simulink model "model"  (R2014a)
settings: Solver=ode45  StartTime=0.0  StopTime=2  RelTol=1e-3
libraries: simulink x3, dspsigattribs x2, dspinverses x1
settings Model: Creator=Lauszus  LastModifiedBy=Lauszus

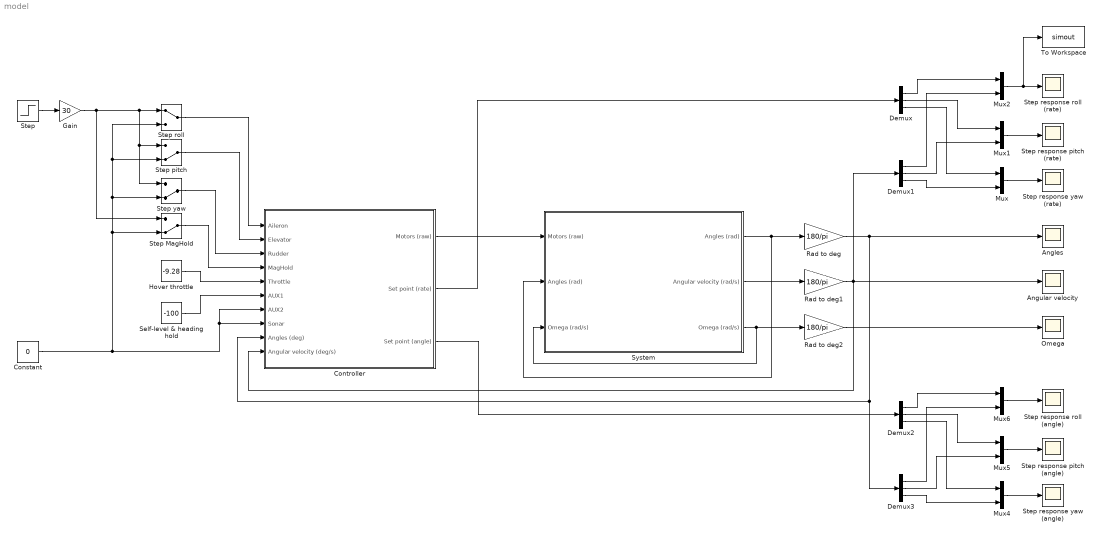
== system model ==
  Angles : Scope
      settings: SaveName=ScopeData2  MaxDataPoints=100000
  Angular velocity : Scope
      settings: MaxDataPoints=100000
  Constant : Constant  Value=0
  Controller : Subsystem
  Demux{,1..3} (4 alike) : Demux  Outputs=3
  Gain : Gain  Gain=30
  Hover throttle : Constant  Value=-9.28
  Mux{,1..2,4..6} (6 alike) : Mux  Inputs=2
  Omega : Scope
      settings: YMin=-2.5  YMax=47.5  SaveName=ScopeData3  MaxDataPoints=100000
  Rad to deg : Gain  Gain=180/pi
  Rad to deg1 : Gain  Gain=180/pi
  Rad to deg2 : Gain  Gain=180/pi
  Self-level & heading hold : Constant  Value=-100
  Step : Step  SampleTime=0
  Step MagHold : ManualSwitch  CurrentSetting=0
  Step pitch : ManualSwitch  CurrentSetting=0
  Step response pitch (angle) : Scope
      settings: SaveName=ScopeData4  MaxDataPoints=100000
  Step response pitch (rate) : Scope
      settings: YMin=46.9  YMax=46.9001  SaveName=ScopeData6  MaxDataPoints=100000
  Step response roll (angle) : Scope
      settings: YMin=44  YMax=48.25  SaveName=ScopeData5  MaxDataPoints=100000
  Step response roll (rate) : Scope
      settings: YMin=44  YMax=48.25  SaveName=ScopeData11  MaxDataPoints=100000
  Step response yaw (angle) : Scope
      settings: YMin=19  YMax=21  SaveName=ScopeData7  MaxDataPoints=100000
  Step response yaw (rate) : Scope
      settings: YMin=19  YMax=21  SaveName=ScopeData10  MaxDataPoints=100000
  Step roll : ManualSwitch
  Step yaw : ManualSwitch  CurrentSetting=0
  System : Subsystem
  To Workspace : ToWorkspace  VariableName=simout  SaveFormat=Timeseries  SampleTime=-1
  wires:
  Self-level & heading hold/1 -> Controller/6(AUX1)
  Constant/1 -> Step MagHold/2, Step pitch/2, Step roll/2, Step yaw/2, Controller/8(Sonar), Controller/7(AUX2)
  Hover throttle/1 -> Controller/5(Throttle)
  System/2(Angular velocity (rad/s)) -> Rad to deg1/1
  Controller/2(Set point (rate)) -> Demux/1
  Step roll/1 -> Controller/1(Aileron)
  Step pitch/1 -> Controller/2(Elevator)
  Mux/1 -> Step response yaw (rate)/1
  Mux1/1 -> Step response pitch (rate)/1
  Mux2/1 -> To Workspace/1, Step response roll (rate)/1
  Demux1/3 -> Mux/2
  Demux/1 -> Mux2/1
  Demux/2 -> Mux1/1
  Demux/3 -> Mux/1
  Demux1/1 -> Mux2/2
  Demux1/2 -> Mux1/2
  Step yaw/1 -> Controller/3(Rudder)
  Step MagHold/1 -> Controller/4(MagHold)
  Step/1 -> Gain/1
  Controller/1(Motors (raw)) -> System/1(Motors (raw))
  System/1(Angles (rad)) -> Rad to deg/1, System/2("Angles (rad) ")
  Gain/1 -> Step yaw/1, Step pitch/1, Step roll/1, Step MagHold/1
  System/3(Omega (rad/s)) -> Rad to deg2/1, System/3("Omega (rad/s) ")
  Rad to deg1/1 -> Controller/10(Angular velocity (deg/s)), Demux1/1, Angular velocity/1
  Rad to deg/1 -> Demux3/1, Controller/9(Angles (deg)), Angles/1
  Rad to deg2/1 -> Omega/1
  Mux5/1 -> Step response pitch (angle)/1
  Mux6/1 -> Step response roll (angle)/1
  Demux3/3 -> Mux4/2
  Demux2/1 -> Mux6/1
  Demux2/2 -> Mux5/1
  Demux2/3 -> Mux4/1
  Demux3/2 -> Mux5/2
  Controller/3(Set point (angle)) -> Demux2/1
  Demux3/1 -> Mux6/2
  Mux4/1 -> Step response yaw (angle)/1

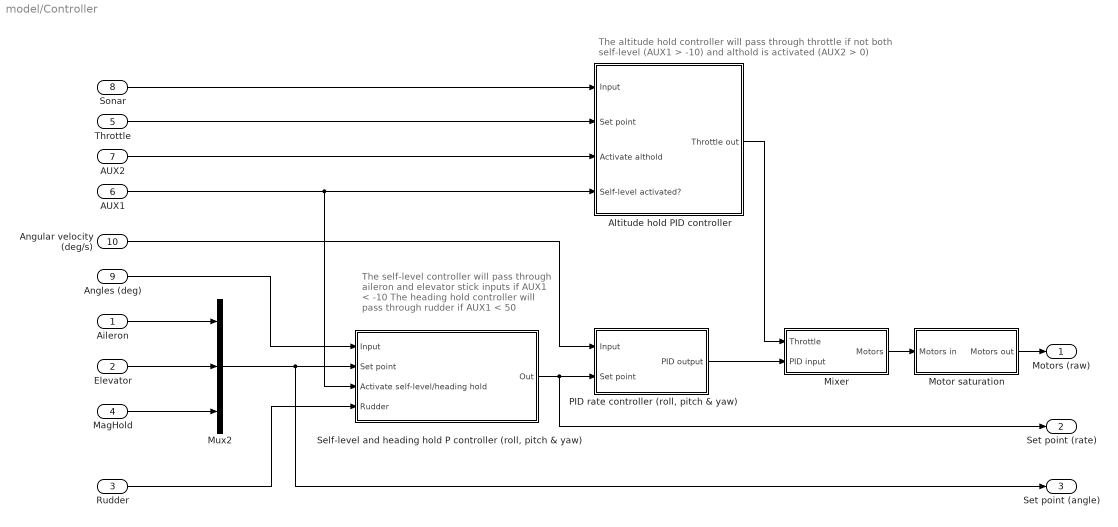
== system model/Controller ==
  note: The self-level controller will pass through aileron and elevator stick inputs if AUX1 < -10
      | The heading hold controller will pass through rudder if AUX1 < 50
  note: The altitude hold controller will pass through throttle if not both
      | self-level (AUX1 > -10) and althold is activated (AUX2 > 0)
  Aileron : Inport
  Elevator : Inport  Port=2
  Rudder : Inport  Port=3
  MagHold : Inport  Port=4
  Throttle : Inport  Port=5
  AUX1 : Inport  Port=6
  AUX2 : Inport  Port=7
  Sonar : Inport  Port=8
  Angles (deg) : Inport  Port=9
  Angular velocity (deg/s) : Inport  Port=10
  Altitude hold PID controller : Subsystem
  Mixer : Subsystem
  Motor saturation : Subsystem
  Mux2 : Mux  Inputs=3
  "PID rate controller (roll, pitch & yaw)" : Subsystem
  "Self-level and heading hold P controller (roll, pitch & yaw)" : Subsystem
  Motors (raw) : Outport
  Set point (rate) : Outport  Port=2
  Set point (angle) : Outport  Port=3
  wires:
  AUX1/1 -> "Self-level and heading hold P controller (roll, pitch & yaw)"/3(Activate self-level/heading hold), Altitude hold PID controller/4(Self-level activated?)
  Angular velocity (deg/s)/1 -> "PID rate controller (roll, pitch & yaw)"/1(Input)
  "Self-level and heading hold P controller (roll, pitch & yaw)"/1(Out) -> "PID rate controller (roll, pitch & yaw)"/2(Set point), Set point (rate)/1
  Sonar/1 -> Altitude hold PID controller/1(Input)
  Throttle/1 -> Altitude hold PID controller/2(Set point)
  AUX2/1 -> Altitude hold PID controller/3(Activate althold)
  Altitude hold PID controller/1(Throttle out) -> Mixer/1(Throttle)
  "PID rate controller (roll, pitch & yaw)"/1(PID output) -> Mixer/2(PID input)
  Mixer/1(Motors) -> Motor saturation/1(Motors in)
  Motor saturation/1(Motors out) -> Motors (raw)/1
  Angles (deg)/1 -> "Self-level and heading hold P controller (roll, pitch & yaw)"/1(Input)
  Aileron/1 -> Mux2/1
  Elevator/1 -> Mux2/2
  Mux2/1 -> Set point (angle)/1, "Self-level and heading hold P controller (roll, pitch & yaw)"/2(Set point)
  MagHold/1 -> Mux2/3
  Rudder/1 -> "Self-level and heading hold P controller (roll, pitch & yaw)"/4(Rudder)

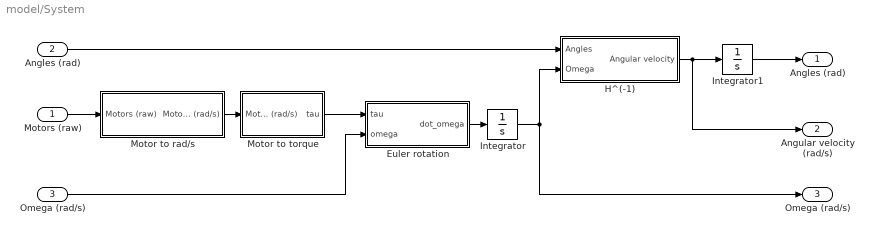
== system model/System ==
  Motors (raw) : Inport
  "Angles (rad) " : Inport  Port=2
  "Omega (rad/s) " : Inport  Port=3
  Euler rotation : Subsystem
  H^(-1) : Subsystem
  Integrator : Integrator
  Integrator1 : Integrator
  Motor to rad/s : Subsystem
  Motor to torque : Subsystem
  Angles (rad) : Outport
  Angular velocity (rad/s) : Outport  Port=2
  Omega (rad/s) : Outport  Port=3
  wires:
  Integrator1/1 -> Angles (rad)/1
  "Angles (rad) "/1 -> H^(-1)/1("Angles ")
  Integrator/1 -> Omega (rad/s)/1, H^(-1)/2(Omega)
  "Omega (rad/s) "/1 -> Euler rotation/2(omega)
  Euler rotation/1(dot_omega) -> Integrator/1
  Motor to torque/1(tau) -> Euler rotation/1(tau)
  Motor to rad/s/1(Motors (rad/s)) -> Motor to torque/1(Motors (rad/s))
  Motors (raw)/1 -> Motor to rad/s/1(Motors (raw))
  H^(-1)/1(Angular velocity) -> Integrator1/1, Angular velocity (rad/s)/1

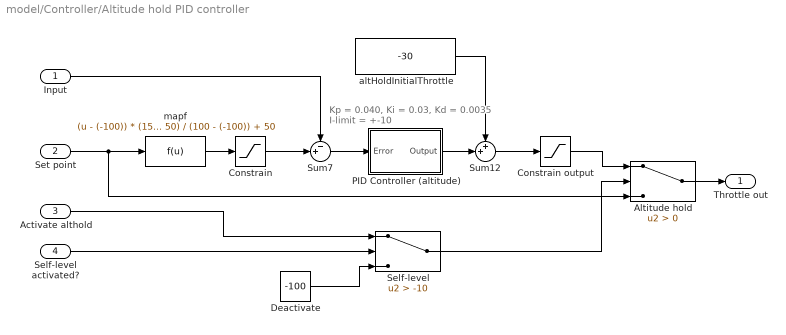
== system model/Controller/Altitude hold PID controller ==
  note: Kp = 0.040, Ki = 0.03, Kd = 0.0035
      | I-limit =  +-10
  Input : Inport
  Set point : Inport  Port=2
  Activate althold : Inport  Port=3
  Self-level activated? : Inport  Port=4
  Altitude hold : Switch  Criteria=u2 > Threshold
  Constrain : Saturate  UpperLimit=1500  LowerLimit=50
  Constrain output : Saturate  UpperLimit=100  LowerLimit=-90
  Deactivate : Constant  Value=-100
  PID Controller (altitude) : Subsystem
  Self-level : Switch  Criteria=u2 > Threshold  Threshold=-10
  Sum12 : Sum  Inputs=++|
  Sum7 : Sum  Inputs=-+|
  altHoldInitialThrottle : Constant  Value=-30
  mapf : Fcn  Expr=(u - (-100)) * (1500 - 50) / (100 - (-100)) + 50
  Throttle out : Outport
  wires:
  Set point/1 -> mapf/1, Altitude hold/3
  Self-level/1 -> Altitude hold/2
  altHoldInitialThrottle/1 -> Sum12/1
  Sum12/1 -> Constrain output/1
  Constrain output/1 -> Altitude hold/1
  Activate althold/1 -> Self-level/1
  Deactivate/1 -> Self-level/3
  Self-level activated?/1 -> Self-level/2
  mapf/1 -> Constrain/1
  Constrain/1 -> Sum7/2
  Input/1 -> Sum7/1
  Altitude hold/1 -> Throttle out/1
  Sum7/1 -> PID Controller (altitude)/1(Error)
  PID Controller (altitude)/1(Output) -> Sum12/2

== system model/Controller/Mixer ==
  note: Motor 1 is bottom right
      | Motor 2 is top right
      | Motor 3 is bottom left
      | Motor 4 is top left
  Throttle : Inport
  PID input : Inport  Port=2
  Demux : Demux  Outputs=3
  Mux1 : Mux
  Sum : Sum  Inputs=+-+-
  Sum1 : Sum  Inputs=+--+
  Sum2 : Sum  Inputs=++++
  Sum3 : Sum  Inputs=++--
  Motors : Outport
  wires:
  Throttle/1 -> Sum3/1, Sum2/1, Sum1/1, Sum/1
  Demux/2 -> Sum/3, Sum1/3, Sum2/3, Sum3/3
  Demux/3 -> Sum/4, Sum1/4, Sum2/4, Sum3/4
  Demux/1 -> Sum3/2, Sum/2, Sum1/2, Sum2/2
  Sum/1 -> Mux1/1
  Sum1/1 -> Mux1/2
  Sum2/1 -> Mux1/3
  Sum3/1 -> Mux1/4
  Mux1/1 -> Motors/1
  PID input/1 -> Demux/1

== system model/Controller/Motor saturation ==
  Motors in : Inport
  If : If  NumInputs=2  IfExpression=u2 > u1
  Max output : Constant  Value=100
  Merge : Merge
  MinMax : MinMax  Function=max
  Passthrough : Subsystem  TreatAsAtomicUnit=on
  Subtract difference : Subsystem  TreatAsAtomicUnit=on
  Sum13 : Sum  Inputs=-+|
  Motors out : Outport
  wires:
  Motors in/1 -> Subtract difference/2(Motors), Passthrough/1(In1), MinMax/1
  If/1 -> Subtract difference/Action
  Subtract difference/1(Out1) -> Merge/1
  If/2 -> Passthrough/Action
  Passthrough/1(Out1) -> Merge/2
  Max output/1 -> Sum13/1, If/1
  MinMax/1 -> If/2, Sum13/2
  Sum13/1 -> Subtract difference/1(Difference)
  Merge/1 -> Motors out/1

== system model/Controller/PID rate controller (roll, pitch & yaw) ==
  note: Kp = 0.310, Ki = 1.65, Kd = 0.00040
      | I-limit =  +-5.85
  note: Kp = 1, Ki = 6, Kd = 0.00040
      | I-limit =  +-10
  note: Kp = 0.310, Ki = 1.65, Kd = 0.00040
      | I-limit =  +-5.85
  Input : Inport
  Set point : Inport  Port=2
  Demux1 : Demux  Outputs=3
  Mux : Mux  Inputs=3
  PID Controller (pitch) : Subsystem
  PID Controller (roll) : Subsystem
  PID Controller (yaw) : Subsystem
  Sum10 : Sum  Inputs=-+|
  PID output : Outport
  wires:
  Mux/1 -> PID output/1
  Set point/1 -> Sum10/2
  Sum10/1 -> Demux1/1
  Input/1 -> Sum10/1
  Demux1/1 -> PID Controller (roll)/1(Error)
  Demux1/2 -> PID Controller (pitch)/1(Error)
  PID Controller (roll)/1(Output) -> Mux/1
  PID Controller (pitch)/1(Output) -> Mux/2
  Demux1/3 -> PID Controller (yaw)/1(Error)
  PID Controller (yaw)/1(Output) -> Mux/3

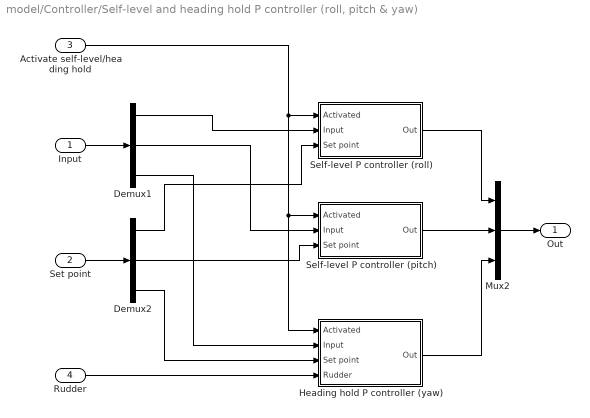
== system model/Controller/Self-level and heading hold P controller (roll, pitch & yaw) ==
  Input : Inport
  Set point : Inport  Port=2
  Activate self-level/heading hold : Inport  Port=3
  Rudder : Inport  Port=4
  Demux1 : Demux  Outputs=3
  Demux2 : Demux  Outputs=3
  Heading hold P controller (yaw) : Subsystem
  Mux2 : Mux  Inputs=3
  Self-level P controller (pitch) : Subsystem
  Self-level P controller (roll) : Subsystem
  Out : Outport
  wires:
  Self-level P controller (roll)/1(Out) -> Mux2/1
  Self-level P controller (pitch)/1(Out) -> Mux2/2
  Input/1 -> Demux1/1
  Set point/1 -> Demux2/1
  Mux2/1 -> Out/1
  Activate self-level/heading hold/1 -> Heading hold P controller (yaw)/1(Activated), Self-level P controller (pitch)/1(Activated), Self-level P controller (roll)/1(Activated)
  Rudder/1 -> Heading hold P controller (yaw)/4(Rudder)
  Heading hold P controller (yaw)/1(Out) -> Mux2/3
  Demux1/1 -> Self-level P controller (roll)/2(Input)
  Demux1/2 -> Self-level P controller (pitch)/2(Input)
  Demux1/3 -> Heading hold P controller (yaw)/2(Input)
  Demux2/1 -> Self-level P controller (roll)/3(Set point)
  Demux2/2 -> Self-level P controller (pitch)/3(Set point)
  Demux2/3 -> Heading hold P controller (yaw)/3(Set point)

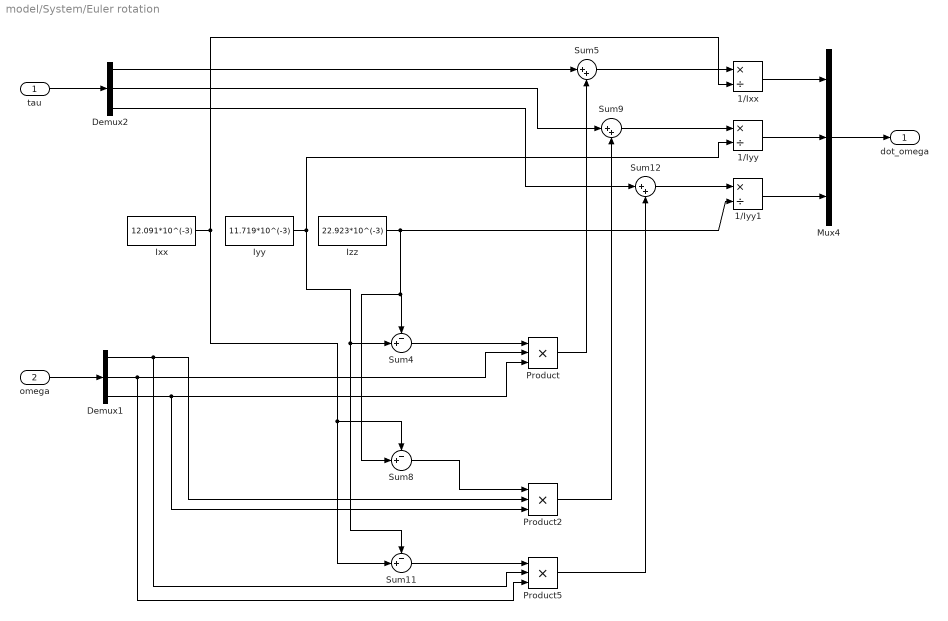
== system model/System/Euler rotation ==
  tau : Inport
  omega : Inport  Port=2
  1/Ixx : Product  Inputs=*/
  1/Iyy : Product  Inputs=*/
  1/Iyy1 : Product  Inputs=*/
  Demux1 : Demux  Outputs=3
  Demux2 : Demux  Outputs=3
  Ixx : Constant  Value=12.091*10^(-3)
  Iyy : Constant  Value=11.719*10^(-3)
  Izz : Constant  Value=22.923*10^(-3)
  Mux4 : Mux  Inputs=3
  Product : Product  Inputs=3
  Product2 : Product  Inputs=3
  Product5 : Product  Inputs=3
  Sum11 : Sum  Inputs=-+|
  Sum12 : Sum  Inputs=|++
  Sum4 : Sum  Inputs=-+|
  Sum5 : Sum  Inputs=|++
  Sum8 : Sum  Inputs=-+|
  Sum9 : Sum  Inputs=|++
  dot_omega : Outport
  wires:
  Iyy/1 -> Sum11/1, Sum4/2, 1/Iyy/2
  Izz/1 -> Sum8/2, Sum4/1, 1/Iyy1/2
  omega/1 -> Demux1/1
  Sum4/1 -> Product/1
  Ixx/1 -> 1/Ixx/2, Sum11/2, Sum8/1
  Sum8/1 -> Product2/1
  Demux1/1 -> Product5/2, Product2/2
  Demux1/2 -> Product5/3, Product/2
  Demux1/3 -> Product2/3, Product/3
  Sum11/1 -> Product5/1
  Mux4/1 -> dot_omega/1
  Sum5/1 -> 1/Ixx/1
  tau/1 -> Demux2/1
  Demux2/1 -> Sum5/1
  Demux2/2 -> Sum9/1
  Demux2/3 -> Sum12/1
  1/Ixx/1 -> Mux4/1
  Sum9/1 -> 1/Iyy/1
  Sum12/1 -> 1/Iyy1/1
  1/Iyy/1 -> Mux4/2
  1/Iyy1/1 -> Mux4/3
  Product/1 -> Sum5/2
  Product2/1 -> Sum9/2
  Product5/1 -> Sum12/2

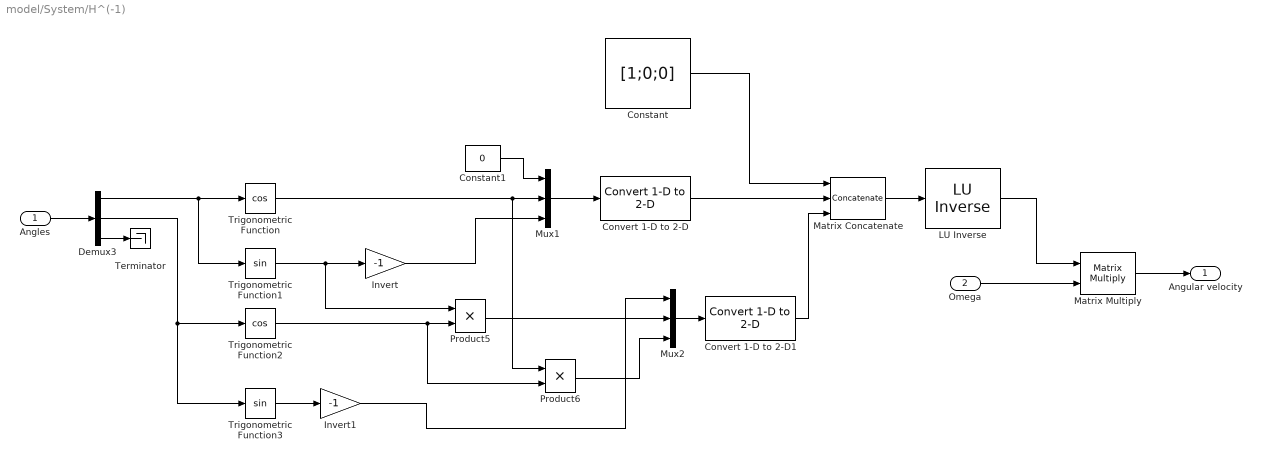
== system model/System/H^(-1) ==
  "Angles " : Inport
  Omega : Inport  Port=2
  " LU Inverse" : dspinverses/ LU Inverse
  Constant : Constant  Value=[1;0;0]  VectorParams1D=off
  Constant1 : Constant  Value=0
  Convert 1-D to 2-D : dspsigattribs/Convert 1-D to 2-D  M=3  N=1  frameBasedOut=off
  Convert 1-D to 2-D1 : dspsigattribs/Convert 1-D to 2-D  M=3  N=1  frameBasedOut=off
  Demux3 : Demux  Outputs=3
  Invert : Gain  Gain=-1
  Invert1 : Gain  Gain=-1
  Matrix Concatenate : Concatenate  NumInputs=3  Mode=Multidimensional array  ConcatenateDimension=2
  Matrix Multiply : Product  Multiplication=Matrix(*)
  Mux1 : Mux  Inputs=3
  Mux2 : Mux  Inputs=3
  Product5 : Product
  Product6 : Product
  Terminator : Terminator
  Trigonometric Function : Trigonometry  Operator=cos
  Trigonometric Function1 : Trigonometry
  Trigonometric Function2 : Trigonometry  Operator=cos
  Trigonometric Function3 : Trigonometry
  Angular velocity : Outport
  wires:
  Constant/1 -> Matrix Concatenate/1
  Constant1/1 -> Mux1/1
  "Angles "/1 -> Demux3/1
  Demux3/1 -> Trigonometric Function1/1, Trigonometric Function/1
  Demux3/2 -> Trigonometric Function2/1, Trigonometric Function3/1
  Trigonometric Function/1 -> Product6/1, Mux1/2
  Trigonometric Function1/1 -> Product5/1, Invert/1
  Invert/1 -> Mux1/3
  Trigonometric Function3/1 -> Invert1/1
  Invert1/1 -> Mux2/1
  Product5/1 -> Mux2/2
  Product6/1 -> Mux2/3
  Trigonometric Function2/1 -> Product5/2, Product6/2
  Mux1/1 -> Convert 1-D to 2-D/1
  Convert 1-D to 2-D/1 -> Matrix Concatenate/2
  Mux2/1 -> Convert 1-D to 2-D1/1
  Convert 1-D to 2-D1/1 -> Matrix Concatenate/3
  Matrix Concatenate/1 -> " LU Inverse"/1
  " LU Inverse"/1 -> Matrix Multiply/1
  Matrix Multiply/1 -> Angular velocity/1
  Omega/1 -> Matrix Multiply/2
  Demux3/3 -> Terminator/1

== system model/System/Motor to rad//s ==
  note: Convert motor out to rad/s
  Motors (raw) : Inport
  Intercept : Constant  Value=677.87
  Slope : Gain  Gain=6.4056
  Sum : Sum  Inputs=++|
  Motors (rad/s) : Outport
  wires:
  Slope/1 -> Sum/2
  Intercept/1 -> Sum/1
  Sum/1 -> Motors (rad/s)/1
  Motors (raw)/1 -> Slope/1

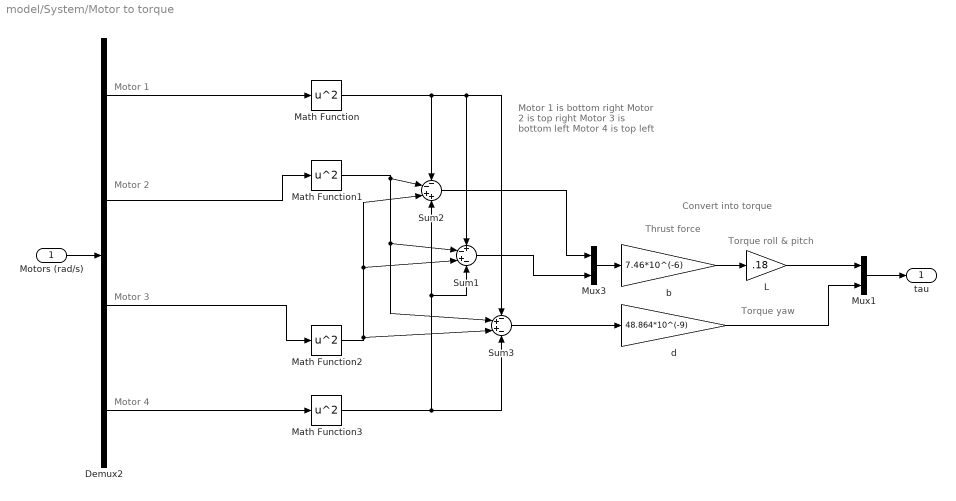
== system model/System/Motor to torque ==
  note: Convert into torque
  note: Motor 1
  note: Motor 1 is bottom right
      | Motor 2 is top right
      | Motor 3 is bottom left
      | Motor 4 is top left
  note: Motor 2
  note: Motor 3
  note: Motor 4
  note: Torque roll & pitch
  note: Thrust force
  note: Torque yaw
  Motors (rad/s) : Inport
  Demux2 : Demux
  L : Gain  Gain=.18
  Math Function{,1..3} (4 alike) : Math  Operator=square  SaturateOnIntegerOverflow=on
  Mux1 : Mux  Inputs=2
  Mux3 : Mux  Inputs=2
  Sum1 : Sum  Inputs=+-+-
  Sum2 : Sum  Inputs=--++
  Sum3 : Sum  Inputs=-++-
  b : Gain  Gain=7.46*10^(-6)
  d : Gain  Gain=48.864*10^(-9)
  tau : Outport
  wires:
  Mux3/1 -> b/1
  Math Function/1 -> Sum3/1, Sum1/1, Sum2/1
  Math Function1/1 -> Sum3/2, Sum1/2, Sum2/2
  Math Function2/1 -> Sum1/3, Sum2/3, Sum3/3
  Sum2/1 -> Mux3/1
  Sum1/1 -> Mux3/2
  Demux2/1 -> Math Function/1
  Demux2/2 -> Math Function1/1
  Demux2/3 -> Math Function2/1
  Demux2/4 -> Math Function3/1
  Sum3/1 -> d/1
  Motors (rad/s)/1 -> Demux2/1
  Math Function3/1 -> Sum3/4, Sum1/4, Sum2/4
  b/1 -> L/1
  L/1 -> Mux1/1
  d/1 -> Mux1/2
  Mux1/1 -> tau/1

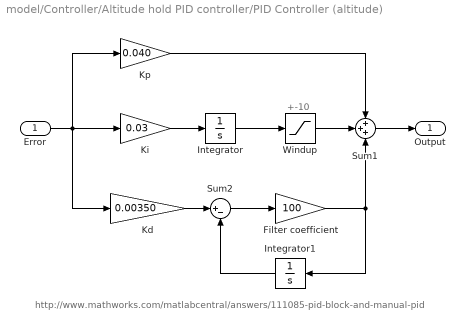
== system model/Controller/Altitude hold PID controller/PID Controller (altitude) ==
  note: http://www.mathworks.com/matlabcentral/answers/111085-pid-block-and-manual-pid
  note: +-10
  Error : Inport
  Filter coefficient : Gain  Gain=100
  Integrator : Integrator
  Integrator1 : Integrator
  Kd : Gain  Gain=0.00350
  Ki : Gain  Gain=0.03
  Kp : Gain  Gain=0.040
  Sum1 : Sum  Inputs=+++
  Sum2 : Sum  Inputs=|+-
  Windup : Saturate  UpperLimit=10  LowerLimit=-10
  Output : Outport
  wires:
  Sum1/1 -> Output/1
  Error/1 -> Ki/1, Kp/1, Kd/1
  Kp/1 -> Sum1/1
  Ki/1 -> Integrator/1
  Integrator/1 -> Windup/1
  Windup/1 -> Sum1/2
  Kd/1 -> Sum2/1
  Sum2/1 -> Filter coefficient/1
  Filter coefficient/1 -> Sum1/3, Integrator1/1
  Integrator1/1 -> Sum2/2

== system model/Controller/Motor saturation/Passthrough ==
  In1 : Inport
  Action Port : ActionPort  ActionType=else
  Out1 : Outport
  wires:
  In1/1 -> Out1/1

== system model/Controller/Motor saturation/Subtract difference ==
  Difference : Inport
  Motors : Inport  Port=2
  Action Port : ActionPort  ActionType=then
  Sum : Sum  Inputs=|+-
  Out1 : Outport
  wires:
  Motors/1 -> Sum/1
  Sum/1 -> Out1/1
  Difference/1 -> Sum/2

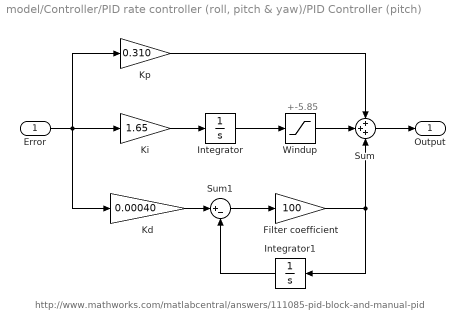
== system model/Controller/PID rate controller (roll, pitch & yaw)/PID Controller (pitch) ==
  note: http://www.mathworks.com/matlabcentral/answers/111085-pid-block-and-manual-pid
  note: +-5.85
  Error : Inport
  Filter coefficient : Gain  Gain=100
  Integrator : Integrator
  Integrator1 : Integrator
  Kd : Gain  Gain=0.00040
  Ki : Gain  Gain=1.65
  Kp : Gain  Gain=0.310
  Sum : Sum  Inputs=+++
  Sum1 : Sum  Inputs=|+-
  Windup : Saturate  UpperLimit=5.85  LowerLimit=-5.85
  Output : Outport
  wires:
  Sum/1 -> Output/1
  Error/1 -> Ki/1, Kp/1, Kd/1
  Kp/1 -> Sum/1
  Ki/1 -> Integrator/1
  Integrator/1 -> Windup/1
  Windup/1 -> Sum/2
  Kd/1 -> Sum1/1
  Sum1/1 -> Filter coefficient/1
  Filter coefficient/1 -> Sum/3, Integrator1/1
  Integrator1/1 -> Sum1/2

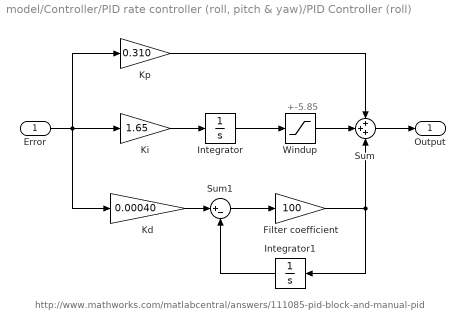
== system model/Controller/PID rate controller (roll, pitch & yaw)/PID Controller (roll) ==
  note: http://www.mathworks.com/matlabcentral/answers/111085-pid-block-and-manual-pid
  note: +-5.85
  Error : Inport
  Filter coefficient : Gain  Gain=100
  Integrator : Integrator
  Integrator1 : Integrator
  Kd : Gain  Gain=0.00040
  Ki : Gain  Gain=1.65
  Kp : Gain  Gain=0.310
  Sum : Sum  Inputs=+++
  Sum1 : Sum  Inputs=|+-
  Windup : Saturate  UpperLimit=5.85  LowerLimit=-5.85
  Output : Outport
  wires:
  Sum/1 -> Output/1
  Error/1 -> Ki/1, Kp/1, Kd/1
  Kp/1 -> Sum/1
  Ki/1 -> Integrator/1
  Integrator/1 -> Windup/1
  Windup/1 -> Sum/2
  Kd/1 -> Sum1/1
  Sum1/1 -> Filter coefficient/1
  Filter coefficient/1 -> Sum/3, Integrator1/1
  Integrator1/1 -> Sum1/2

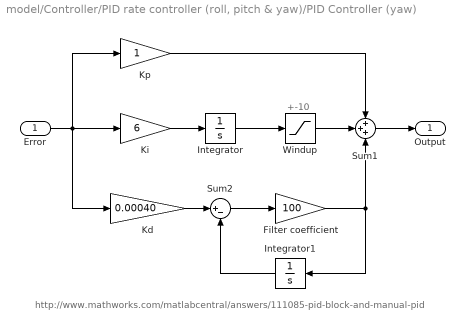
== system model/Controller/PID rate controller (roll, pitch & yaw)/PID Controller (yaw) ==
  note: http://www.mathworks.com/matlabcentral/answers/111085-pid-block-and-manual-pid
  note: +-10
  Error : Inport
  Filter coefficient : Gain  Gain=100
  Integrator : Integrator
  Integrator1 : Integrator
  Kd : Gain  Gain=0.00040
  Ki : Gain  Gain=6
  Kp : Gain
  Sum1 : Sum  Inputs=+++
  Sum2 : Sum  Inputs=|+-
  Windup : Saturate  UpperLimit=10  LowerLimit=-10
  Output : Outport
  wires:
  Sum1/1 -> Output/1
  Error/1 -> Ki/1, Kp/1, Kd/1
  Kp/1 -> Sum1/1
  Ki/1 -> Integrator/1
  Integrator/1 -> Windup/1
  Windup/1 -> Sum1/2
  Kd/1 -> Sum2/1
  Sum2/1 -> Filter coefficient/1
  Filter coefficient/1 -> Sum1/3, Integrator1/1
  Integrator1/1 -> Sum2/2

== system model/Controller/Self-level and heading hold P controller (roll, pitch & yaw)/Heading hold P controller (yaw) ==
  note: Kp = 0.65
  Activated : Inport
  Input : Inport  Port=2
  Set point : Inport  Port=3
  Rudder : Inport  Port=4
  Heading hold? : Switch  Criteria=u2 > Threshold  Threshold=50
  P Controller (heading) : simulink/Continuous/PID Controller  Controller=P  TimeDomain=Continuous-time  SampleTime=1  IntegratorMethod=Forward Euler  FilterMethod=Forward Euler  Form=Parallel  P=0.65  I=1  D=0  N=100  InitialConditionSource=internal  InitialConditionForIntegrator=0  InitialConditionForFilter=0  ExternalReset=none  LimitOutput=off  UpperSaturationLimit=inf  LowerSaturationLimit=-inf  LinearizeAsGain=on  AntiWindupMode=none  Kb=1  TrackingMode=off  Kt=1  PParamMin=[]  PParamMax=[]  IParamMin=[]  IParamMax=[]  DParamMin=[]  DParamMax=[]  NParamMin=[]  NParamMax=[]  KbParamMin=[]  KbParamMax=[]  KtParamMin=[]  KtParamMax=[]  POutMin=[]  POutMax=[]  IOutMin=[]  IOutMax=[]  DOutMin=[]  DOutMax=[]  NOutMin=[]  NOutMax=[]  KbOutMin=[]  KbOutMax=[]  KtOutMin=[]  KtOutMax=[]  IntegratorOutMin=[]  IntegratorOutMax=[]  FilterOutMin=[]  FilterOutMax=[]  SumOutMin=[]  SumOutMax=[]  SumI1OutMin=[]  SumI1OutMax=[]  SumI2OutMin=[]  SumI2OutMax=[]  SumI3OutMin=[]  SumI3OutMax=[]  SumDOutMin=[]  SumDOutMax=[]  SaturationOutMin=[]  SaturationOutMax=[]  IntegratorContinuousStateAttributes=''  IntegratorStateMustResolveToSignalObject=off  IntegratorRTWStateStorageClass=Auto  FilterContinuousStateAttributes=''  FilterStateMustResolveToSignalObject=off  FilterRTWStateStorageClass=Auto
  Stick scaling yaw : Gain  Gain=2
  Sum11 : Sum  Inputs=|++
  Sum6 : Sum  Inputs=-+|
  Out : Outport
  wires:
  Set point/1 -> Sum6/2
  Stick scaling yaw/1 -> Out/1
  Heading hold?/1 -> Stick scaling yaw/1
  Sum6/1 -> P Controller (heading)/1
  P Controller (heading)/1 -> Sum11/1
  Sum11/1 -> Heading hold?/1
  Rudder/1 -> Sum11/2, Heading hold?/3
  Input/1 -> Sum6/1
  Activated/1 -> Heading hold?/2

== system model/Controller/Self-level and heading hold P controller (roll, pitch & yaw)/Self-level P controller (pitch) ==
  note: Kp = 4.5
  Activated : Inport
  Input : Inport  Port=2
  Set point : Inport  Port=3
  "Constrain angle " : Saturate  UpperLimit=50  LowerLimit=-50
  P Controller (self-level pitch) : simulink/Continuous/PID Controller  Controller=P  TimeDomain=Continuous-time  SampleTime=1  IntegratorMethod=Forward Euler  FilterMethod=Forward Euler  Form=Parallel  P=4.50  I=1  D=0  N=100  InitialConditionSource=internal  InitialConditionForIntegrator=0  InitialConditionForFilter=0  ExternalReset=none  LimitOutput=off  UpperSaturationLimit=inf  LowerSaturationLimit=-inf  LinearizeAsGain=on  AntiWindupMode=none  Kb=1  TrackingMode=off  Kt=1  PParamMin=[]  PParamMax=[]  IParamMin=[]  IParamMax=[]  DParamMin=[]  DParamMax=[]  NParamMin=[]  NParamMax=[]  KbParamMin=[]  KbParamMax=[]  KtParamMin=[]  KtParamMax=[]  POutMin=[]  POutMax=[]  IOutMin=[]  IOutMax=[]  DOutMin=[]  DOutMax=[]  NOutMin=[]  NOutMax=[]  KbOutMin=[]  KbOutMax=[]  KtOutMin=[]  KtOutMax=[]  IntegratorOutMin=[]  IntegratorOutMax=[]  FilterOutMin=[]  FilterOutMax=[]  SumOutMin=[]  SumOutMax=[]  SumI1OutMin=[]  SumI1OutMax=[]  SumI2OutMin=[]  SumI2OutMax=[]  SumI3OutMin=[]  SumI3OutMax=[]  SumDOutMin=[]  SumDOutMax=[]  SaturationOutMin=[]  SaturationOutMax=[]  IntegratorContinuousStateAttributes=''  IntegratorStateMustResolveToSignalObject=off  IntegratorRTWStateStorageClass=Auto  FilterContinuousStateAttributes=''  FilterStateMustResolveToSignalObject=off  FilterRTWStateStorageClass=Auto
  Self-level (pitch)? : Switch  Criteria=u2 > Threshold  Threshold=-10
  Stick scaling pitch : Gain  Gain=4.69
  Sum5 : Sum  Inputs=-+|
  Out : Outport
  wires:
  Set point/1 -> Stick scaling pitch/1, "Constrain angle "/1
  Self-level (pitch)?/1 -> Out/1
  P Controller (self-level pitch)/1 -> Self-level (pitch)?/1
  Sum5/1 -> P Controller (self-level pitch)/1
  "Constrain angle "/1 -> Sum5/2
  Stick scaling pitch/1 -> Self-level (pitch)?/3
  Input/1 -> Sum5/1
  Activated/1 -> Self-level (pitch)?/2

== system model/Controller/Self-level and heading hold P controller (roll, pitch & yaw)/Self-level P controller (roll) ==
  note: Kp = 4.5
  Activated : Inport
  Input : Inport  Port=2
  Set point : Inport  Port=3
  Constrain angle : Saturate  UpperLimit=50  LowerLimit=-50
  P Controller (self-level roll) : simulink/Continuous/PID Controller  Controller=P  TimeDomain=Continuous-time  SampleTime=1  IntegratorMethod=Forward Euler  FilterMethod=Forward Euler  Form=Parallel  P=4.50  I=1  D=0  N=100  InitialConditionSource=internal  InitialConditionForIntegrator=0  InitialConditionForFilter=0  ExternalReset=none  LimitOutput=off  UpperSaturationLimit=inf  LowerSaturationLimit=-inf  LinearizeAsGain=on  AntiWindupMode=none  Kb=1  TrackingMode=off  Kt=1  PParamMin=[]  PParamMax=[]  IParamMin=[]  IParamMax=[]  DParamMin=[]  DParamMax=[]  NParamMin=[]  NParamMax=[]  KbParamMin=[]  KbParamMax=[]  KtParamMin=[]  KtParamMax=[]  POutMin=[]  POutMax=[]  IOutMin=[]  IOutMax=[]  DOutMin=[]  DOutMax=[]  NOutMin=[]  NOutMax=[]  KbOutMin=[]  KbOutMax=[]  KtOutMin=[]  KtOutMax=[]  IntegratorOutMin=[]  IntegratorOutMax=[]  FilterOutMin=[]  FilterOutMax=[]  SumOutMin=[]  SumOutMax=[]  SumI1OutMin=[]  SumI1OutMax=[]  SumI2OutMin=[]  SumI2OutMax=[]  SumI3OutMin=[]  SumI3OutMax=[]  SumDOutMin=[]  SumDOutMax=[]  SaturationOutMin=[]  SaturationOutMax=[]  IntegratorContinuousStateAttributes=''  IntegratorStateMustResolveToSignalObject=off  IntegratorRTWStateStorageClass=Auto  FilterContinuousStateAttributes=''  FilterStateMustResolveToSignalObject=off  FilterRTWStateStorageClass=Auto
  Self-level (roll)? : Switch  Criteria=u2 > Threshold  Threshold=-10
  Stick scaling roll : Gain  Gain=4.69
  Sum4 : Sum  Inputs=-+|
  Out : Outport
  wires:
  Set point/1 -> Stick scaling roll/1, Constrain angle/1
  Sum4/1 -> P Controller (self-level roll)/1
  Constrain angle/1 -> Sum4/2
  Activated/1 -> Self-level (roll)?/2
  P Controller (self-level roll)/1 -> Self-level (roll)?/1
  Stick scaling roll/1 -> Self-level (roll)?/3
  Input/1 -> Sum4/1
  Self-level (roll)?/1 -> Out/1
